simulink subsystem "Motor_d"  (R2024b)
settings: Solver=VariableStepAuto  StartTime=0.0  StopTime=10.0  RelTol=1e-3
undefined symbols (not defined in the file): DiscIntNeverNeededParam, motor, wheels
settings Model: Creator=Marij  LastModifiedBy=marijn

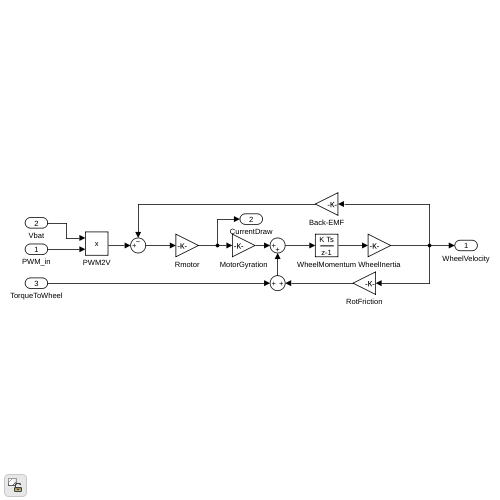
[thumbnail: Simulink's stored preview of the top-level diagram]
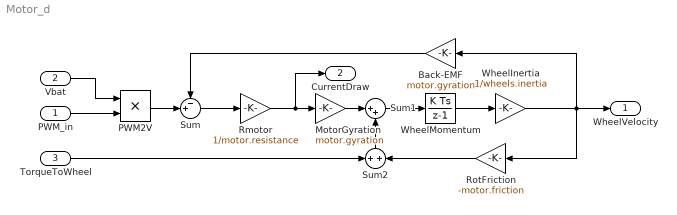
== system Motor_d ==
  PWM_in : Inport
  Vbat : Inport  Port=2
  TorqueToWheel : Inport  Port=3
  Back-EMF : Gain  Gain=motor.gyration
  MotorGyration : Gain  Gain=motor.gyration
  PWM2V : Product
  Rmotor : Gain  Gain=1/motor.resistance
  RotFriction : Gain  Gain=-motor.friction
  Sum : Sum  Inputs=-+|
  Sum1 : Sum  Inputs=|++
  Sum2 : Sum  Inputs=+|+
  WheelInertia : Gain  Gain=1/wheels.inertia
  WheelMomentum : DiscreteIntegrator  SampleTime=0.0100000000000000002  ICPrevOutput=DiscIntNeverNeededParam  ICPrevScaledInput=DiscIntNeverNeededParam  mask(DiscretizedDiscreteIntegrator){}
      mask init:
      | %zoh
  WheelVelocity : Outport  Unit=rad/s
  CurrentDraw : Outport  Port=2  Unit=A  PortDimensions=1
  wires:
  Rmotor/1 -> CurrentDraw/1, MotorGyration/1
  Sum1/1 -> WheelMomentum/1
  PWM_in/1 -> PWM2V/2
  Sum/1 -> Rmotor/1
  MotorGyration/1 -> Sum1/1
  PWM2V/1 -> Sum/2
  Vbat/1 -> PWM2V/1
  Back-EMF/1 -> Sum/1
  WheelInertia/1 -> WheelVelocity/1, Back-EMF/1, RotFriction/1
  WheelMomentum/1 -> WheelInertia/1
  RotFriction/1 -> Sum2/2
  TorqueToWheel/1 -> Sum2/1
  Sum2/1 -> Sum1/2
